simulink model "library"  (R2013a)
settings: Solver=ode45  StartTime=0.0  StopTime=10.0  RelTol=1e-3
settings Model: Creator=admin  LastModifiedBy=admin

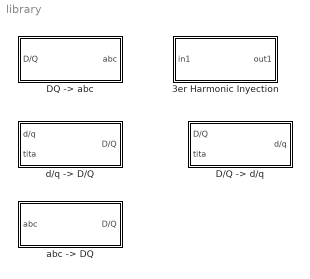
== system library ==
  3er Harmonic Inyection : Subsystem
  "D/Q -> d/q" : Subsystem
  "DQ -> abc" : Subsystem
  "abc -> DQ " : Subsystem
  "d/q -> D/Q " : Subsystem

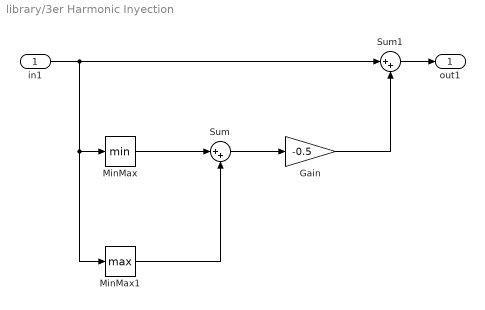
== system library/3er Harmonic Inyection ==
  in1 : Inport
  Gain : Gain  Gain=-0.5
  MinMax : MinMax
  MinMax1 : MinMax  Function=max
  Sum : Sum  Inputs=|++
  Sum1 : Sum  Inputs=|++
  out1 : Outport
  wires:
  in1/1 -> Sum1/1, MinMax1/1, MinMax/1
  MinMax/1 -> Sum/1
  MinMax1/1 -> Sum/2
  Sum1/1 -> out1/1
  Sum/1 -> Gain/1
  Gain/1 -> Sum1/2

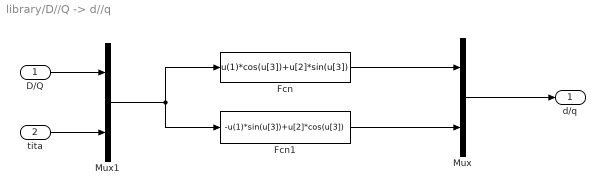
== system library/D//Q -> d//q ==
  D/Q : Inport
  tita : Inport  Port=2
  Fcn : Fcn  Expr=u(1)*cos(u[3])+u[2]*sin(u[3])
  Fcn1 : Fcn  Expr=-u(1)*sin(u[3])+u[2]*cos(u[3])
  Mux : Mux  Inputs=2
  Mux1 : Mux  Inputs=2
  d/q : Outport
  wires:
  Mux/1 -> d/q/1
  Fcn/1 -> Mux/1
  Fcn1/1 -> Mux/2
  D/Q/1 -> Mux1/1
  tita/1 -> Mux1/2
  Mux1/1 -> Fcn/1, Fcn1/1

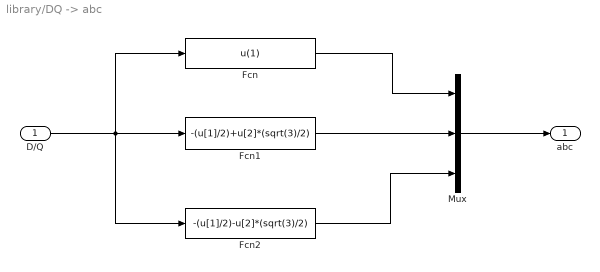
== system library/DQ -> abc ==
  D/Q : Inport
  Fcn : Fcn  Expr=u(1)
  Fcn1 : Fcn  Expr=-(u[1]/2)+u[2]*(sqrt(3)/2)
  Fcn2 : Fcn  Expr=-(u[1]/2)-u[2]*(sqrt(3)/2)
  Mux : Mux  Inputs=3
  abc : Outport
  wires:
  Mux/1 -> abc/1
  D/Q/1 -> Fcn2/1, Fcn1/1, Fcn/1
  Fcn/1 -> Mux/1
  Fcn1/1 -> Mux/2
  Fcn2/1 -> Mux/3

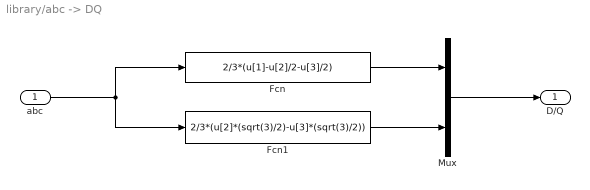
== system library/abc -> DQ  ==
  abc : Inport
  Fcn : Fcn  Expr=2/3*(u[1]-u[2]/2-u[3]/2)
  Fcn1 : Fcn  Expr=2/3*(u[2]*(sqrt(3)/2)-u[3]*(sqrt(3)/2))
  Mux : Mux  Inputs=2
  D/Q : Outport
  wires:
  Mux/1 -> D/Q/1
  abc/1 -> Fcn1/1, Fcn/1
  Fcn/1 -> Mux/1
  Fcn1/1 -> Mux/2

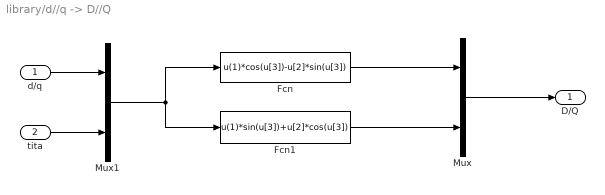
== system library/d//q -> D//Q  ==
  d/q : Inport
  tita : Inport  Port=2
  Fcn : Fcn  Expr=u(1)*cos(u[3])-u[2]*sin(u[3])
  Fcn1 : Fcn  Expr=u(1)*sin(u[3])+u[2]*cos(u[3])
  Mux : Mux  Inputs=2
  Mux1 : Mux  Inputs=2
  D/Q : Outport
  wires:
  Mux/1 -> D/Q/1
  Fcn/1 -> Mux/1
  Fcn1/1 -> Mux/2
  d/q/1 -> Mux1/1
  tita/1 -> Mux1/2
  Mux1/1 -> Fcn/1, Fcn1/1
